simulink model "Article1_half_a_trial"  (R2016a)
settings: Solver=VariableStepAuto  StartTime=0.0  StopTime=10.0  RelTol=1e-3
libraries: elec_lib x9
settings Model: Creator=syf  LastModifiedBy=syf

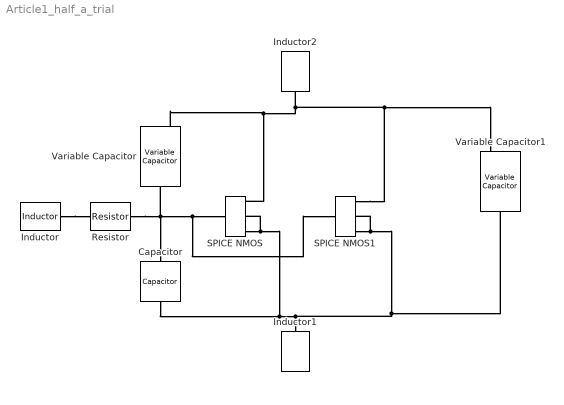
== system Article1_half_a_trial ==
  Capacitor : elec_lib/Passive Devices/Capacitor  enable_table=0  c=1e-6 F  Cvec=[ 1e-5 1e-6 ] F  Vvec=[ 0 10 ] V  CV_table_symmetry=1  C_tol=5  enable_C_tol=0  tol_distribution=1  nSigma=4  r=1e-6 Ohm  g=0 1/Ohm  initV=0 V  enable_operating_limits=0  operating_limit_action=1  max_working_voltage_range=[ -25 25 ] V  power_rating=1 W  enable_faults=0  fault_action=1  Cscale_faulted=100  R_faulted=0.001 Ohm  G_faulted=0 1/Ohm  tau_fault=0.001 s  enable_temporal_fault=0  t_fault=1 s  enable_behavioral_fault=0  max_permissible_voltage_range=[ -100 100 ] V  t_fail_on_voltage=1 s
  Inductor : elec_lib/Passive Devices/Inductor  l=1e-6 H  L_tol=20  enable_L_tol=0  tol_distribution=1  nSigma=4  r=0 Ohm  g=1e-9 1/Ohm  initI=0 A  enable_operating_limits=0  operating_limit_action=1  max_working_current=1 A  power_rating=1 W  enable_faults=0  fault_action=1  lambdaPercent=50  k_faulted=0.9999 Ohm  turnsShort=0  openCct=0  groundShort=0  groundShortG=0 1/Ohm  tau_fault=0.001 s  enable_temporal_fault=0  t_fault=1 s  enable_behavioral_fault=0  max_permissible_voltage=100 V  n_fail_on_voltage=1  max_permissible_current=1 A  t_fail_on_current=1 s
  Inductor1 : elec_lib/Passive Devices/Inductor  l=1e-6 H  L_tol=20  enable_L_tol=0  tol_distribution=1  nSigma=4  r=0 Ohm  g=1e-9 1/Ohm  initI=0 A  enable_operating_limits=0  operating_limit_action=1  max_working_current=1 A  power_rating=1 W  enable_faults=0  fault_action=1  lambdaPercent=50  k_faulted=0.9999 Ohm  turnsShort=0  openCct=0  groundShort=0  groundShortG=0 1/Ohm  tau_fault=0.001 s  enable_temporal_fault=0  t_fault=1 s  enable_behavioral_fault=0  max_permissible_voltage=100 V  n_fail_on_voltage=1  max_permissible_current=1 A  t_fail_on_current=1 s
  Inductor2 : elec_lib/Passive Devices/Inductor  l=1e-6 H  L_tol=20  enable_L_tol=0  tol_distribution=1  nSigma=4  r=0 Ohm  g=1e-9 1/Ohm  initI=0 A  enable_operating_limits=0  operating_limit_action=1  max_working_current=1 A  power_rating=1 W  enable_faults=0  fault_action=1  lambdaPercent=50  k_faulted=0.9999 Ohm  turnsShort=0  openCct=0  groundShort=0  groundShortG=0 1/Ohm  tau_fault=0.001 s  enable_temporal_fault=0  t_fault=1 s  enable_behavioral_fault=0  max_permissible_voltage=100 V  n_fail_on_voltage=1  max_permissible_current=1 A  t_fail_on_current=1 s
  Resistor : elec_lib/Passive Devices/Resistor  R=1 Ohm  R_tol=5  enable_R_tol=0  tol_distribution=1  nSigma=4  enable_operating_limits=0  operating_limit_action=2  max_working_voltage=100 V  power_rating=1 W  enable_faults=0  fault_action=1  R_faulted=Inf Ohm  enable_temporal_fault=0  t_fault=1 s  enable_behavioral_fault=0  max_permissible_current=1 A  t_fail_on_current=1 s  noise_mode=0  sample_time=0.001 s  repeatability=1  auto_seed=3917579146  user_seed=0  Tdevice=25 degC  alpha=0.00393 1/K  Tmeas=25 degC  thermal_mass=100 J/K  initial_temperature=25 degC  power_derating_T1=70 degC  power_derating_T2=155 degC  operating_temperature_range_vec=[ -50 150 ] degC
  SPICE NMOS : elec_lib/Additional Components/SPICE-Compatible Components/Semiconductor Devices/SPICE NMOS  AREA=1  SCALE=1  LENGTH=1e-4 m  WIDTH=1e-4 m  AD=0 m^2  AS=0 m^2  PD=0 m  PS=0 m  NRD=1  NRS=1  LEVEL=1  VTO=0 V  KP=2e-5 A/V^2  GAMMA=0 V^0.50000  PHI=0.6 V  LAMBDA=0 1/V  RD=0.01 Ohm  RS=1e-4 Ohm  C_param=1  CBD=0 F  CBS=0 F  IS=1e-14 A  ND=1  PB=0.8 V  CGSO=0 F/m  CGDO=0 F/m  CGBO=0 F/m  RSH=NaN Ohm  CJ=0 F/m^2  MJ=0.5  CJSW=0 F/m  MJSW=0.5  JS=0 A/m^2  TOX=NaN m  LD=0 m  U0=600 cm^2/s/V  FC=0.5  NSUB=NaN 1/cm^3  TPG=1  NSS=0 1/cm^2  UEXP=0  UCRIT=1e+4 V/cm  NEFF=1  DELTA=0  VMAX=0 m/s  XJ=0 m  NFS=0 1/cm^2  ETA=0  THETA=0 1/V  KAPPA=0.2  T_param=1  TOFFSET=0 K  TFIXED=300.15 K  TMEAS=300.15 K  IC_given=1  ICVDS=0 V  ICVGS=0 V  ICVBS=0 V  MTYPE=1
  SPICE NMOS1 : elec_lib/Additional Components/SPICE-Compatible Components/Semiconductor Devices/SPICE NMOS  AREA=1  SCALE=1  LENGTH=1e-4 m  WIDTH=1e-4 m  AD=0 m^2  AS=0 m^2  PD=0 m  PS=0 m  NRD=1  NRS=1  LEVEL=1  VTO=0 V  KP=2e-5 A/V^2  GAMMA=0 V^0.50000  PHI=0.6 V  LAMBDA=0 1/V  RD=0.01 Ohm  RS=1e-4 Ohm  C_param=1  CBD=0 F  CBS=0 F  IS=1e-14 A  ND=1  PB=0.8 V  CGSO=0 F/m  CGDO=0 F/m  CGBO=0 F/m  RSH=NaN Ohm  CJ=0 F/m^2  MJ=0.5  CJSW=0 F/m  MJSW=0.5  JS=0 A/m^2  TOX=NaN m  LD=0 m  U0=600 cm^2/s/V  FC=0.5  NSUB=NaN 1/cm^3  TPG=1  NSS=0 1/cm^2  UEXP=0  UCRIT=1e+4 V/cm  NEFF=1  DELTA=0  VMAX=0 m/s  XJ=0 m  NFS=0 1/cm^2  ETA=0  THETA=0 1/V  KAPPA=0.2  T_param=1  TOFFSET=0 K  TFIXED=300.15 K  TMEAS=300.15 K  IC_given=1  ICVDS=0 V  ICVGS=0 V  ICVBS=0 V  MTYPE=1
  Variable Capacitor : elec_lib/Passive Devices/Variable Capacitor  prm=2  Cmin=1e-9 F  r=1e-6 Ohm  v0=0 V  q0=0 c
  Variable Capacitor1 : elec_lib/Passive Devices/Variable Capacitor  prm=2  Cmin=1e-9 F  r=1e-6 Ohm  v0=0 V  q0=0 c
  connections:
  Resistor/RConn1 -- Variable Capacitor/RConn1 -- Capacitor/LConn1 -- SPICE NMOS1/LConn1 -- SPICE NMOS/LConn1
  Inductor/RConn1 -- Resistor/LConn1
  Capacitor/RConn1 -- SPICE NMOS/RConn2 -- SPICE NMOS/RConn3 -- Variable Capacitor1/RConn1 -- SPICE NMOS1/RConn2 -- SPICE NMOS1/RConn3 -- Inductor1/LConn1
  Variable Capacitor/LConn2 -- SPICE NMOS1/RConn1 -- Variable Capacitor1/LConn2 -- Inductor2/RConn1 -- SPICE NMOS/RConn1
